simulink model "Lotka_Volterra"  (R2023a)
settings: Solver=VariableStepAuto  StartTime=0.0  StopTime=100.0  RelTol=1e-3
settings Model: Creator=pc  LastModifiedBy=pc
settings DataIOCC: ReturnWorkspaceOutputs=off  TimeSaveName=t

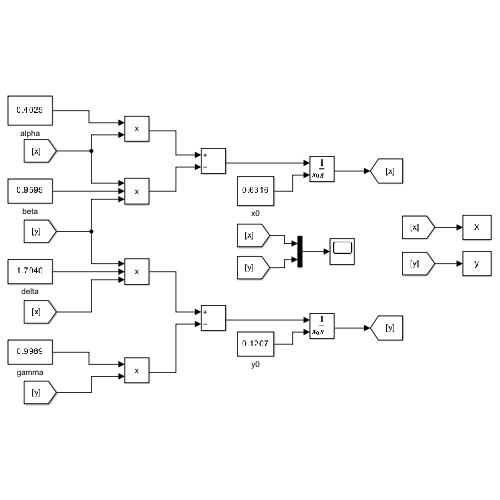
[thumbnail: Simulink's stored preview of the top-level diagram]
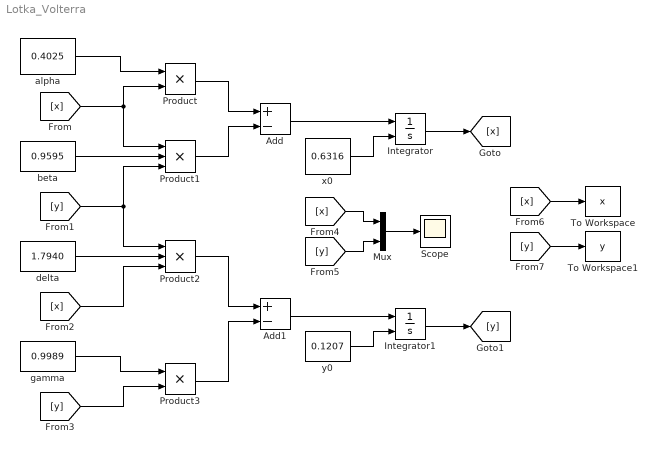
== system Lotka_Volterra ==
  Add : Sum  Inputs=+-
  Add1 : Sum  Inputs=+-
  Integrator : Integrator  InitialConditionSource=external
  Integrator1 : Integrator  InitialConditionSource=external
  Mux : Mux  Inputs=2
  Product : Product
  Product1 : Product  Inputs=3
  Product2 : Product  Inputs=3
  Product3 : Product
  Scope : Scope
  To Workspace : ToWorkspace  VariableName=x  SampleTime=-1
  To Workspace1 : ToWorkspace  VariableName=y  SampleTime=-1
  alpha : Constant  Value=0.4025
  beta : Constant  Value=0.9595
  delta : Constant  Value=1.7940
  gamma : Constant  Value=0.9989
  x0 : Constant  Value=0.6316
  y0 : Constant  Value=0.1207
  wires:
  x0/1 -> Integrator/2
  y0/1 -> Integrator1/2
  Integrator/1 -> [x]
  Integrator1/1 -> [y]
  alpha/1 -> Product/1
  [x] -> Product1/1, Product/2
  beta/1 -> Product1/2
  [y] -> Product2/1, Product1/3
  delta/1 -> Product2/2
  [x] -> Product2/3
  gamma/1 -> Product3/1
  [y] -> Product3/2
  Product/1 -> Add/1
  Product1/1 -> Add/2
  Product2/1 -> Add1/1
  Product3/1 -> Add1/2
  Add1/1 -> Integrator1/1
  Add/1 -> Integrator/1
  Mux/1 -> Scope/1
  [y] -> Mux/2
  [x] -> Mux/1
  [x] -> To Workspace/1
  [y] -> To Workspace1/1
